simulink model "Simulation_v2"  (R2020a)
settings: Solver=VariableStepAuto  StartTime=0.0  StopTime=tmax  RelTol=1e-3
values from neighbouring files (symbols this model uses):
  BPden = [1 alpha]    [RunSimulation.m]    (also in RunTest.m)
  BPnum = [0.3 alpha]    [RunSimulation.m]    (also in RunTest.m)
  c = 250    [RunSimulation.m]    (also in RunTest.m)
  fc = 0.45    [RunTest.m]
  Ft = 360000    [RunTest.m]
  l = 18    [RunSimulation.m]    (also in RunTest.m)
  num_wagons = 10    [RunTest.m]
  p0 = 0    [RunSimulation.m]    (also in RunTest.m)
  pool = readmatrix('pool.csv')    [RunTest.m]
  Pres = 0/1000*[5.7/771 0 1.6]    [RunSimulation.m]    (also in RunTest.m)
  RBD = 5    [RunSimulation.m]    (also in RunTest.m)
  tl = .1    (= 0.1)    [RunSimulation.m]    (also in RunTest.m)
  trackgradient = 0    [RunTest.m]
  v0 = 100/3.6    (= 27.7777777778)    [RunSimulation.m]
  VBD = 3.5    [RunSimulation.m]    (also in RunTest.m)
libraries: simulink x43, commrandsrc3 x40
(part 2 of 4)

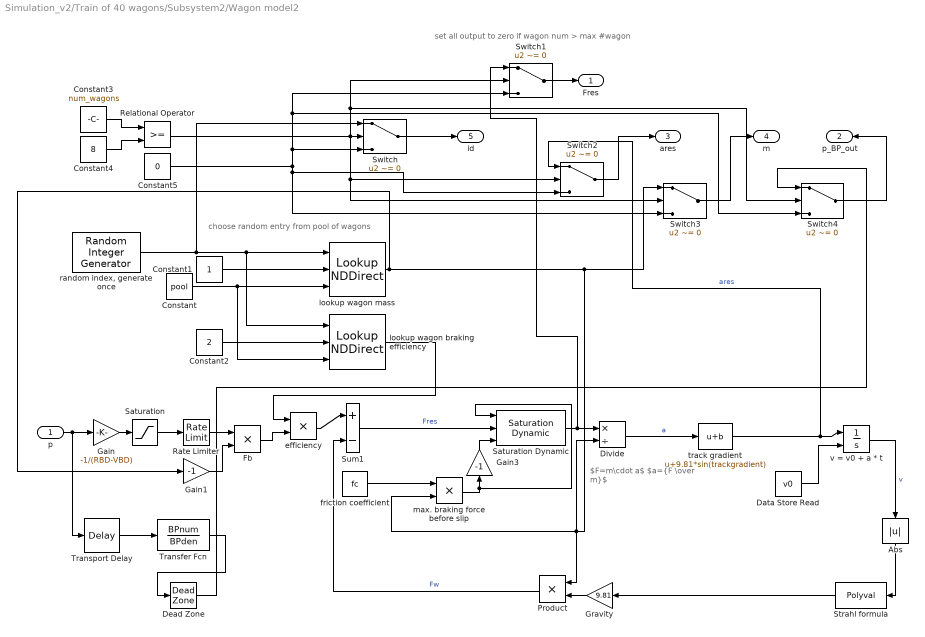
== system Simulation_v2/Train of 40 wagons/Subsystem2/Wagon model2 ==
  note: set all output to zero if wagon num > max #wagon
  note: choose random entry from pool of wagons
  note: $F=m\cdot a$ $a={F \over m}$
  p : Inport
  Abs : Abs
  Constant : Constant  Value=pool
  Constant1 : Constant
  Constant2 : Constant  Value=2
  Constant3 : Constant  Value=num_wagons
  Constant4 : Constant  Value=8
  Constant5 : Constant  Value=0  OutDataTypeStr=uint32
  Data Store Read : DataStoreRead  DataStoreName=v0
  Dead Zone : DeadZone  LowerValue=-0.005  UpperValue=0.005  SaturateOnIntegerOverflow=on
  Divide : Product  Inputs=*/
  Fb : Product  Inputs=**
  Gain : Gain  Gain=-1/(RBD-VBD)
  Gain1 : Gain  Gain=-1
  Gain3 : Gain  Gain=-1
  Gravity : Gain  Gain=9.81
  Product : Product
  Rate Limiter : RateLimiter  RisingSlewLimit=1/tf  FallingSlewLimit=-1/tl  SampleTimeMode=inherited
  Relational Operator : RelationalOperator  OutDataTypeStr=boolean  RndMeth=Simplest
  Saturation : Saturate  UpperLimit=1  LowerLimit=0
  Saturation Dynamic : simulink/Discontinuities/Saturation Dynamic  OutMin=[]  OutMax=[]  OutDataTypeStr=Inherit: Same as second input  OutDataType=fixdt(1, 16)  OutScaling=2^-10  DoSatur=off
  Strahl formula : Polyval  Coefs=Pres
  Sum1 : Sum  Inputs=|+-
  Switch{,1..4} (5 alike) : Switch  Criteria=u2 ~= 0
  Transfer Fcn : TransferFcn  Numerator=BPnum  Denominator=BPden
  Transport Delay : TransportDelay  DelayTime=l/c  InitialOutput=p0
  efficiency : Product  Inputs=**
  friction coefficient : Constant  Value=fc
  lookup wagon braking efficiency : LookupNDDirect  TableIsInput=on
  lookup wagon mass : LookupNDDirect  TableIsInput=on
  max. braking force before slip : Product  Inputs=**
  "random index, generate once " : commrandsrc3/Random Integer Generator  SetSize=500  SeedSource=Auto  Seed=0  SampleTime=999999  SamplesPerFrame=1  OutputDataType=uint32  SimulateUsing=Interpreted execution
  track gradient : Bias  Bias=9.81*sin(trackgradient)
  v = v0 + a * t : Integrator  InitialConditionSource=external  InitialCondition=v0
  Fres : Outport  VectorParamsAs1DForOutWhenUnconnected=off
  p_BP_out : Outport  Port=2  VectorParamsAs1DForOutWhenUnconnected=off
  ares : Outport  Port=3
  m : Outport  Port=4
  "id " : Outport  Port=5
  wires:
  Strahl formula/1 -> Gravity/1
  Abs/1 -> Strahl formula/1
  Gravity/1 -> Product/2
  Product/1 -> Sum1/2  "Fw"
  v = v0 + a * t/1 -> Abs/1  "v"
  lookup wagon mass/1 -> Gain1/1, Switch3/1, max. braking force before slip/2, Divide/2, Product/1
  Divide/1 -> track gradient/1  "a"
  Gain/1 -> Saturation/1
  Fb/1 -> efficiency/2
  Saturation/1 -> Rate Limiter/1
  Rate Limiter/1 -> Fb/1
  Transfer Fcn/1 -> Dead Zone/1
  Transport Delay/1 -> Transfer Fcn/1
  efficiency/1 -> Sum1/1
  track gradient/1 -> Switch2/1, v = v0 + a * t/1  "ares"
  p/1 -> Gain/1, Transport Delay/1
  friction coefficient/1 -> max. braking force before slip/1
  Sum1/1 -> Saturation Dynamic/2  "Fres"
  Saturation Dynamic/1 -> Switch1/1, Divide/1
  max. braking force before slip/1 -> Saturation Dynamic/1, Gain3/1
  Gain3/1 -> Saturation Dynamic/3
  Data Store Read/1 -> v = v0 + a * t/2
  Dead Zone/1 -> Switch4/1
  Constant/1 -> lookup wagon braking efficiency/3, lookup wagon mass/3
  "random index, generate once "/1 -> Switch/1, lookup wagon mass/1, lookup wagon braking efficiency/1
  Constant1/1 -> lookup wagon mass/2
  Constant2/1 -> lookup wagon braking efficiency/2
  lookup wagon braking efficiency/1 -> efficiency/1
  Gain1/1 -> Fb/2
  Constant3/1 -> Relational Operator/1
  Constant4/1 -> Relational Operator/2
  Relational Operator/1 -> Switch1/2, Switch4/2, Switch2/2, Switch3/2, Switch/2
  Switch/1 -> "id "/1
  Constant5/1 -> Switch4/3, Switch1/3, Switch/3, Switch2/3, Switch3/3
  Switch1/1 -> Fres/1
  Switch2/1 -> ares/1
  Switch3/1 -> m/1
  Switch4/1 -> p_BP_out/1

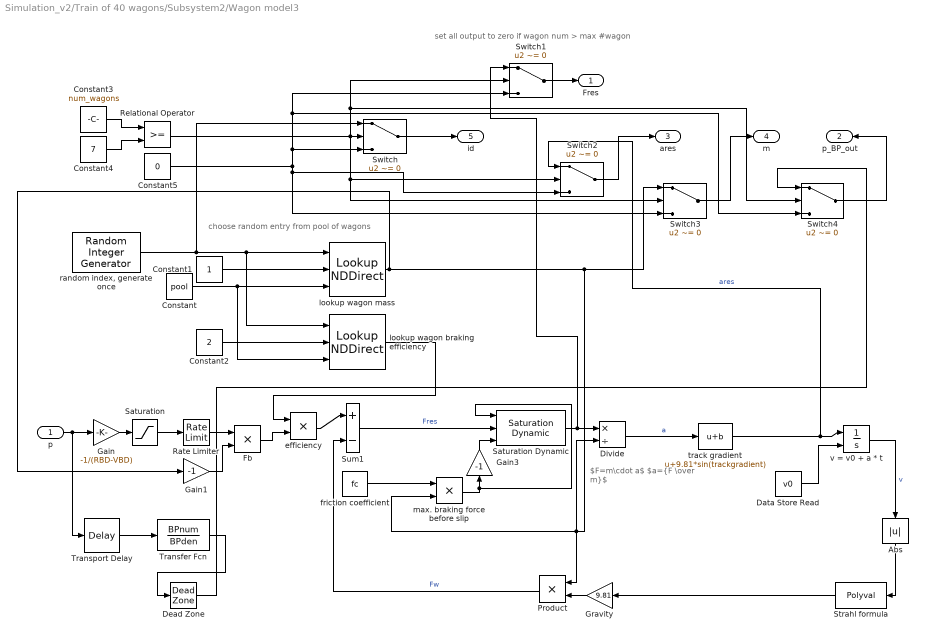
== system Simulation_v2/Train of 40 wagons/Subsystem2/Wagon model3 ==
  note: set all output to zero if wagon num > max #wagon
  note: choose random entry from pool of wagons
  note: $F=m\cdot a$ $a={F \over m}$
  p : Inport
  Abs : Abs
  Constant : Constant  Value=pool
  Constant1 : Constant
  Constant2 : Constant  Value=2
  Constant3 : Constant  Value=num_wagons
  Constant4 : Constant  Value=7
  Constant5 : Constant  Value=0  OutDataTypeStr=uint32
  Data Store Read : DataStoreRead  DataStoreName=v0
  Dead Zone : DeadZone  LowerValue=-0.005  UpperValue=0.005  SaturateOnIntegerOverflow=on
  Divide : Product  Inputs=*/
  Fb : Product  Inputs=**
  Gain : Gain  Gain=-1/(RBD-VBD)
  Gain1 : Gain  Gain=-1
  Gain3 : Gain  Gain=-1
  Gravity : Gain  Gain=9.81
  Product : Product
  Rate Limiter : RateLimiter  RisingSlewLimit=1/tf  FallingSlewLimit=-1/tl  SampleTimeMode=inherited
  Relational Operator : RelationalOperator  OutDataTypeStr=boolean  RndMeth=Simplest
  Saturation : Saturate  UpperLimit=1  LowerLimit=0
  Saturation Dynamic : simulink/Discontinuities/Saturation Dynamic  OutMin=[]  OutMax=[]  OutDataTypeStr=Inherit: Same as second input  OutDataType=fixdt(1, 16)  OutScaling=2^-10  DoSatur=off
  Strahl formula : Polyval  Coefs=Pres
  Sum1 : Sum  Inputs=|+-
  Switch{,1..4} (5 alike) : Switch  Criteria=u2 ~= 0
  Transfer Fcn : TransferFcn  Numerator=BPnum  Denominator=BPden
  Transport Delay : TransportDelay  DelayTime=l/c  InitialOutput=p0
  efficiency : Product  Inputs=**
  friction coefficient : Constant  Value=fc
  lookup wagon braking efficiency : LookupNDDirect  TableIsInput=on
  lookup wagon mass : LookupNDDirect  TableIsInput=on
  max. braking force before slip : Product  Inputs=**
  "random index, generate once " : commrandsrc3/Random Integer Generator  SetSize=500  SeedSource=Auto  Seed=0  SampleTime=999999  SamplesPerFrame=1  OutputDataType=uint32  SimulateUsing=Interpreted execution
  track gradient : Bias  Bias=9.81*sin(trackgradient)
  v = v0 + a * t : Integrator  InitialConditionSource=external  InitialCondition=v0
  Fres : Outport  VectorParamsAs1DForOutWhenUnconnected=off
  p_BP_out : Outport  Port=2  VectorParamsAs1DForOutWhenUnconnected=off
  ares : Outport  Port=3
  m : Outport  Port=4
  "id " : Outport  Port=5
  wires:
  Strahl formula/1 -> Gravity/1
  Abs/1 -> Strahl formula/1
  Gravity/1 -> Product/2
  Product/1 -> Sum1/2  "Fw"
  v = v0 + a * t/1 -> Abs/1  "v"
  lookup wagon mass/1 -> Gain1/1, Switch3/1, max. braking force before slip/2, Divide/2, Product/1
  Divide/1 -> track gradient/1  "a"
  Gain/1 -> Saturation/1
  Fb/1 -> efficiency/2
  Saturation/1 -> Rate Limiter/1
  Rate Limiter/1 -> Fb/1
  Transfer Fcn/1 -> Dead Zone/1
  Transport Delay/1 -> Transfer Fcn/1
  efficiency/1 -> Sum1/1
  track gradient/1 -> Switch2/1, v = v0 + a * t/1  "ares"
  p/1 -> Gain/1, Transport Delay/1
  friction coefficient/1 -> max. braking force before slip/1
  Sum1/1 -> Saturation Dynamic/2  "Fres"
  Saturation Dynamic/1 -> Switch1/1, Divide/1
  max. braking force before slip/1 -> Saturation Dynamic/1, Gain3/1
  Gain3/1 -> Saturation Dynamic/3
  Data Store Read/1 -> v = v0 + a * t/2
  Dead Zone/1 -> Switch4/1
  Constant/1 -> lookup wagon braking efficiency/3, lookup wagon mass/3
  "random index, generate once "/1 -> Switch/1, lookup wagon mass/1, lookup wagon braking efficiency/1
  Constant1/1 -> lookup wagon mass/2
  Constant2/1 -> lookup wagon braking efficiency/2
  lookup wagon braking efficiency/1 -> efficiency/1
  Gain1/1 -> Fb/2
  Constant3/1 -> Relational Operator/1
  Constant4/1 -> Relational Operator/2
  Relational Operator/1 -> Switch1/2, Switch4/2, Switch2/2, Switch3/2, Switch/2
  Switch/1 -> "id "/1
  Constant5/1 -> Switch4/3, Switch1/3, Switch/3, Switch2/3, Switch3/3
  Switch1/1 -> Fres/1
  Switch2/1 -> ares/1
  Switch3/1 -> m/1
  Switch4/1 -> p_BP_out/1

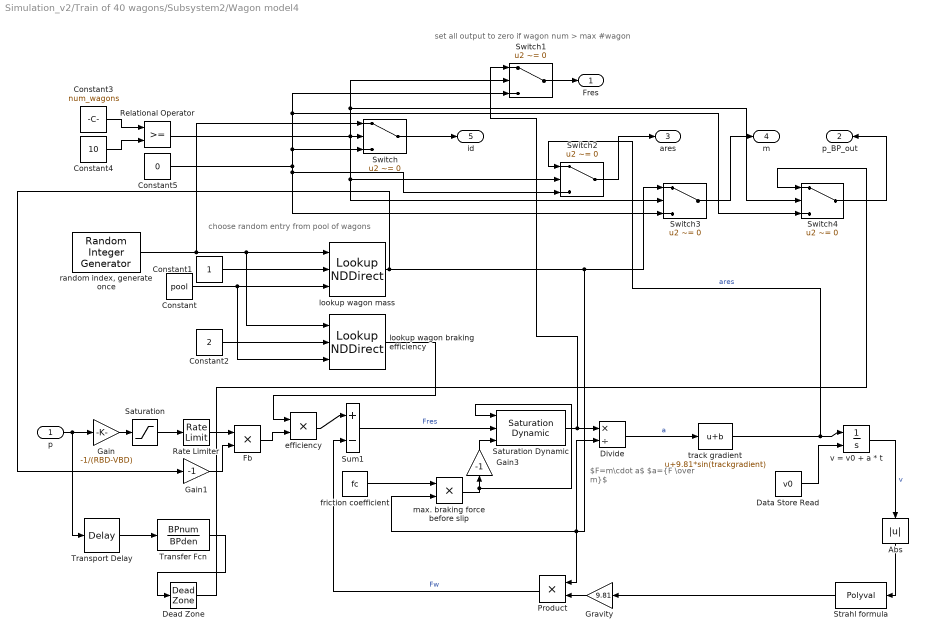
== system Simulation_v2/Train of 40 wagons/Subsystem2/Wagon model4 ==
  note: set all output to zero if wagon num > max #wagon
  note: choose random entry from pool of wagons
  note: $F=m\cdot a$ $a={F \over m}$
  p : Inport
  Abs : Abs
  Constant : Constant  Value=pool
  Constant1 : Constant
  Constant2 : Constant  Value=2
  Constant3 : Constant  Value=num_wagons
  Constant4 : Constant  Value=10
  Constant5 : Constant  Value=0  OutDataTypeStr=uint32
  Data Store Read : DataStoreRead  DataStoreName=v0
  Dead Zone : DeadZone  LowerValue=-0.005  UpperValue=0.005  SaturateOnIntegerOverflow=on
  Divide : Product  Inputs=*/
  Fb : Product  Inputs=**
  Gain : Gain  Gain=-1/(RBD-VBD)
  Gain1 : Gain  Gain=-1
  Gain3 : Gain  Gain=-1
  Gravity : Gain  Gain=9.81
  Product : Product
  Rate Limiter : RateLimiter  RisingSlewLimit=1/tf  FallingSlewLimit=-1/tl  SampleTimeMode=inherited
  Relational Operator : RelationalOperator  OutDataTypeStr=boolean  RndMeth=Simplest
  Saturation : Saturate  UpperLimit=1  LowerLimit=0
  Saturation Dynamic : simulink/Discontinuities/Saturation Dynamic  OutMin=[]  OutMax=[]  OutDataTypeStr=Inherit: Same as second input  OutDataType=fixdt(1, 16)  OutScaling=2^-10  DoSatur=off
  Strahl formula : Polyval  Coefs=Pres
  Sum1 : Sum  Inputs=|+-
  Switch{,1..4} (5 alike) : Switch  Criteria=u2 ~= 0
  Transfer Fcn : TransferFcn  Numerator=BPnum  Denominator=BPden
  Transport Delay : TransportDelay  DelayTime=l/c  InitialOutput=p0
  efficiency : Product  Inputs=**
  friction coefficient : Constant  Value=fc
  lookup wagon braking efficiency : LookupNDDirect  TableIsInput=on
  lookup wagon mass : LookupNDDirect  TableIsInput=on
  max. braking force before slip : Product  Inputs=**
  "random index, generate once " : commrandsrc3/Random Integer Generator  SetSize=500  SeedSource=Auto  Seed=0  SampleTime=999999  SamplesPerFrame=1  OutputDataType=uint32  SimulateUsing=Interpreted execution
  track gradient : Bias  Bias=9.81*sin(trackgradient)
  v = v0 + a * t : Integrator  InitialConditionSource=external  InitialCondition=v0
  Fres : Outport  VectorParamsAs1DForOutWhenUnconnected=off
  p_BP_out : Outport  Port=2  VectorParamsAs1DForOutWhenUnconnected=off
  ares : Outport  Port=3
  m : Outport  Port=4
  "id " : Outport  Port=5
  wires:
  Strahl formula/1 -> Gravity/1
  Abs/1 -> Strahl formula/1
  Gravity/1 -> Product/2
  Product/1 -> Sum1/2  "Fw"
  v = v0 + a * t/1 -> Abs/1  "v"
  lookup wagon mass/1 -> Gain1/1, Switch3/1, max. braking force before slip/2, Divide/2, Product/1
  Divide/1 -> track gradient/1  "a"
  Gain/1 -> Saturation/1
  Fb/1 -> efficiency/2
  Saturation/1 -> Rate Limiter/1
  Rate Limiter/1 -> Fb/1
  Transfer Fcn/1 -> Dead Zone/1
  Transport Delay/1 -> Transfer Fcn/1
  efficiency/1 -> Sum1/1
  track gradient/1 -> Switch2/1, v = v0 + a * t/1  "ares"
  p/1 -> Gain/1, Transport Delay/1
  friction coefficient/1 -> max. braking force before slip/1
  Sum1/1 -> Saturation Dynamic/2  "Fres"
  Saturation Dynamic/1 -> Switch1/1, Divide/1
  max. braking force before slip/1 -> Saturation Dynamic/1, Gain3/1
  Gain3/1 -> Saturation Dynamic/3
  Data Store Read/1 -> v = v0 + a * t/2
  Dead Zone/1 -> Switch4/1
  Constant/1 -> lookup wagon braking efficiency/3, lookup wagon mass/3
  "random index, generate once "/1 -> Switch/1, lookup wagon mass/1, lookup wagon braking efficiency/1
  Constant1/1 -> lookup wagon mass/2
  Constant2/1 -> lookup wagon braking efficiency/2
  lookup wagon braking efficiency/1 -> efficiency/1
  Gain1/1 -> Fb/2
  Constant3/1 -> Relational Operator/1
  Constant4/1 -> Relational Operator/2
  Relational Operator/1 -> Switch1/2, Switch4/2, Switch2/2, Switch3/2, Switch/2
  Switch/1 -> "id "/1
  Constant5/1 -> Switch4/3, Switch1/3, Switch/3, Switch2/3, Switch3/3
  Switch1/1 -> Fres/1
  Switch2/1 -> ares/1
  Switch3/1 -> m/1
  Switch4/1 -> p_BP_out/1

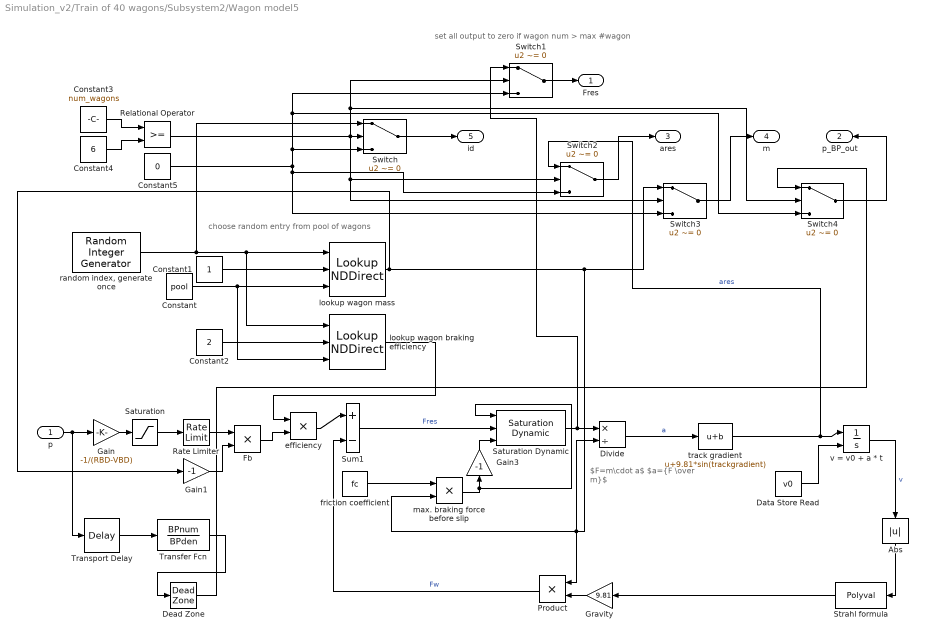
== system Simulation_v2/Train of 40 wagons/Subsystem2/Wagon model5 ==
  note: set all output to zero if wagon num > max #wagon
  note: choose random entry from pool of wagons
  note: $F=m\cdot a$ $a={F \over m}$
  p : Inport
  Abs : Abs
  Constant : Constant  Value=pool
  Constant1 : Constant
  Constant2 : Constant  Value=2
  Constant3 : Constant  Value=num_wagons
  Constant4 : Constant  Value=6
  Constant5 : Constant  Value=0  OutDataTypeStr=uint32
  Data Store Read : DataStoreRead  DataStoreName=v0
  Dead Zone : DeadZone  LowerValue=-0.005  UpperValue=0.005  SaturateOnIntegerOverflow=on
  Divide : Product  Inputs=*/
  Fb : Product  Inputs=**
  Gain : Gain  Gain=-1/(RBD-VBD)
  Gain1 : Gain  Gain=-1
  Gain3 : Gain  Gain=-1
  Gravity : Gain  Gain=9.81
  Product : Product
  Rate Limiter : RateLimiter  RisingSlewLimit=1/tf  FallingSlewLimit=-1/tl  SampleTimeMode=inherited
  Relational Operator : RelationalOperator  OutDataTypeStr=boolean  RndMeth=Simplest
  Saturation : Saturate  UpperLimit=1  LowerLimit=0
  Saturation Dynamic : simulink/Discontinuities/Saturation Dynamic  OutMin=[]  OutMax=[]  OutDataTypeStr=Inherit: Same as second input  OutDataType=fixdt(1, 16)  OutScaling=2^-10  DoSatur=off
  Strahl formula : Polyval  Coefs=Pres
  Sum1 : Sum  Inputs=|+-
  Switch{,1..4} (5 alike) : Switch  Criteria=u2 ~= 0
  Transfer Fcn : TransferFcn  Numerator=BPnum  Denominator=BPden
  Transport Delay : TransportDelay  DelayTime=l/c  InitialOutput=p0
  efficiency : Product  Inputs=**
  friction coefficient : Constant  Value=fc
  lookup wagon braking efficiency : LookupNDDirect  TableIsInput=on
  lookup wagon mass : LookupNDDirect  TableIsInput=on
  max. braking force before slip : Product  Inputs=**
  "random index, generate once " : commrandsrc3/Random Integer Generator  SetSize=500  SeedSource=Auto  Seed=0  SampleTime=999999  SamplesPerFrame=1  OutputDataType=uint32  SimulateUsing=Interpreted execution
  track gradient : Bias  Bias=9.81*sin(trackgradient)
  v = v0 + a * t : Integrator  InitialConditionSource=external  InitialCondition=v0
  Fres : Outport  VectorParamsAs1DForOutWhenUnconnected=off
  p_BP_out : Outport  Port=2  VectorParamsAs1DForOutWhenUnconnected=off
  ares : Outport  Port=3
  m : Outport  Port=4
  "id " : Outport  Port=5
  wires:
  Strahl formula/1 -> Gravity/1
  Abs/1 -> Strahl formula/1
  Gravity/1 -> Product/2
  Product/1 -> Sum1/2  "Fw"
  v = v0 + a * t/1 -> Abs/1  "v"
  lookup wagon mass/1 -> Gain1/1, Switch3/1, max. braking force before slip/2, Divide/2, Product/1
  Divide/1 -> track gradient/1  "a"
  Gain/1 -> Saturation/1
  Fb/1 -> efficiency/2
  Saturation/1 -> Rate Limiter/1
  Rate Limiter/1 -> Fb/1
  Transfer Fcn/1 -> Dead Zone/1
  Transport Delay/1 -> Transfer Fcn/1
  efficiency/1 -> Sum1/1
  track gradient/1 -> Switch2/1, v = v0 + a * t/1  "ares"
  p/1 -> Gain/1, Transport Delay/1
  friction coefficient/1 -> max. braking force before slip/1
  Sum1/1 -> Saturation Dynamic/2  "Fres"
  Saturation Dynamic/1 -> Switch1/1, Divide/1
  max. braking force before slip/1 -> Saturation Dynamic/1, Gain3/1
  Gain3/1 -> Saturation Dynamic/3
  Data Store Read/1 -> v = v0 + a * t/2
  Dead Zone/1 -> Switch4/1
  Constant/1 -> lookup wagon braking efficiency/3, lookup wagon mass/3
  "random index, generate once "/1 -> Switch/1, lookup wagon mass/1, lookup wagon braking efficiency/1
  Constant1/1 -> lookup wagon mass/2
  Constant2/1 -> lookup wagon braking efficiency/2
  lookup wagon braking efficiency/1 -> efficiency/1
  Gain1/1 -> Fb/2
  Constant3/1 -> Relational Operator/1
  Constant4/1 -> Relational Operator/2
  Relational Operator/1 -> Switch1/2, Switch4/2, Switch2/2, Switch3/2, Switch/2
  Switch/1 -> "id "/1
  Constant5/1 -> Switch4/3, Switch1/3, Switch/3, Switch2/3, Switch3/3
  Switch1/1 -> Fres/1
  Switch2/1 -> ares/1
  Switch3/1 -> m/1
  Switch4/1 -> p_BP_out/1

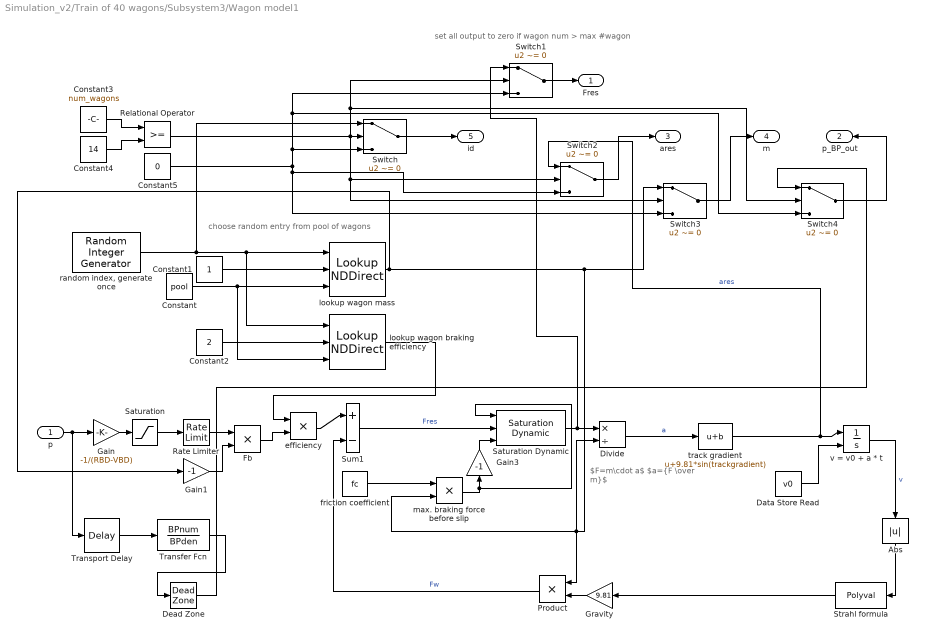
== system Simulation_v2/Train of 40 wagons/Subsystem3/Wagon model1 ==
  note: set all output to zero if wagon num > max #wagon
  note: choose random entry from pool of wagons
  note: $F=m\cdot a$ $a={F \over m}$
  p : Inport
  Abs : Abs
  Constant : Constant  Value=pool
  Constant1 : Constant
  Constant2 : Constant  Value=2
  Constant3 : Constant  Value=num_wagons
  Constant4 : Constant  Value=14
  Constant5 : Constant  Value=0  OutDataTypeStr=uint32
  Data Store Read : DataStoreRead  DataStoreName=v0
  Dead Zone : DeadZone  LowerValue=-0.005  UpperValue=0.005  SaturateOnIntegerOverflow=on
  Divide : Product  Inputs=*/
  Fb : Product  Inputs=**
  Gain : Gain  Gain=-1/(RBD-VBD)
  Gain1 : Gain  Gain=-1
  Gain3 : Gain  Gain=-1
  Gravity : Gain  Gain=9.81
  Product : Product
  Rate Limiter : RateLimiter  RisingSlewLimit=1/tf  FallingSlewLimit=-1/tl  SampleTimeMode=inherited
  Relational Operator : RelationalOperator  OutDataTypeStr=boolean  RndMeth=Simplest
  Saturation : Saturate  UpperLimit=1  LowerLimit=0
  Saturation Dynamic : simulink/Discontinuities/Saturation Dynamic  OutMin=[]  OutMax=[]  OutDataTypeStr=Inherit: Same as second input  OutDataType=fixdt(1, 16)  OutScaling=2^-10  DoSatur=off
  Strahl formula : Polyval  Coefs=Pres
  Sum1 : Sum  Inputs=|+-
  Switch{,1..4} (5 alike) : Switch  Criteria=u2 ~= 0
  Transfer Fcn : TransferFcn  Numerator=BPnum  Denominator=BPden
  Transport Delay : TransportDelay  DelayTime=l/c  InitialOutput=p0
  efficiency : Product  Inputs=**
  friction coefficient : Constant  Value=fc
  lookup wagon braking efficiency : LookupNDDirect  TableIsInput=on
  lookup wagon mass : LookupNDDirect  TableIsInput=on
  max. braking force before slip : Product  Inputs=**
  "random index, generate once " : commrandsrc3/Random Integer Generator  SetSize=500  SeedSource=Auto  Seed=0  SampleTime=999999  SamplesPerFrame=1  OutputDataType=uint32  SimulateUsing=Interpreted execution
  track gradient : Bias  Bias=9.81*sin(trackgradient)
  v = v0 + a * t : Integrator  InitialConditionSource=external  InitialCondition=v0
  Fres : Outport  VectorParamsAs1DForOutWhenUnconnected=off
  p_BP_out : Outport  Port=2  VectorParamsAs1DForOutWhenUnconnected=off
  ares : Outport  Port=3
  m : Outport  Port=4
  "id " : Outport  Port=5
  wires:
  Strahl formula/1 -> Gravity/1
  Abs/1 -> Strahl formula/1
  Gravity/1 -> Product/2
  Product/1 -> Sum1/2  "Fw"
  v = v0 + a * t/1 -> Abs/1  "v"
  lookup wagon mass/1 -> Gain1/1, Switch3/1, max. braking force before slip/2, Divide/2, Product/1
  Divide/1 -> track gradient/1  "a"
  Gain/1 -> Saturation/1
  Fb/1 -> efficiency/2
  Saturation/1 -> Rate Limiter/1
  Rate Limiter/1 -> Fb/1
  Transfer Fcn/1 -> Dead Zone/1
  Transport Delay/1 -> Transfer Fcn/1
  efficiency/1 -> Sum1/1
  track gradient/1 -> Switch2/1, v = v0 + a * t/1  "ares"
  p/1 -> Gain/1, Transport Delay/1
  friction coefficient/1 -> max. braking force before slip/1
  Sum1/1 -> Saturation Dynamic/2  "Fres"
  Saturation Dynamic/1 -> Switch1/1, Divide/1
  max. braking force before slip/1 -> Saturation Dynamic/1, Gain3/1
  Gain3/1 -> Saturation Dynamic/3
  Data Store Read/1 -> v = v0 + a * t/2
  Dead Zone/1 -> Switch4/1
  Constant/1 -> lookup wagon braking efficiency/3, lookup wagon mass/3
  "random index, generate once "/1 -> Switch/1, lookup wagon mass/1, lookup wagon braking efficiency/1
  Constant1/1 -> lookup wagon mass/2
  Constant2/1 -> lookup wagon braking efficiency/2
  lookup wagon braking efficiency/1 -> efficiency/1
  Gain1/1 -> Fb/2
  Constant3/1 -> Relational Operator/1
  Constant4/1 -> Relational Operator/2
  Relational Operator/1 -> Switch1/2, Switch4/2, Switch2/2, Switch3/2, Switch/2
  Switch/1 -> "id "/1
  Constant5/1 -> Switch4/3, Switch1/3, Switch/3, Switch2/3, Switch3/3
  Switch1/1 -> Fres/1
  Switch2/1 -> ares/1
  Switch3/1 -> m/1
  Switch4/1 -> p_BP_out/1

== system Simulation_v2/Train of 40 wagons/Subsystem3/Wagon model2 ==
  note: set all output to zero if wagon num > max #wagon
  note: choose random entry from pool of wagons
  note: $F=m\cdot a$ $a={F \over m}$
  p : Inport
  Abs : Abs
  Constant : Constant  Value=pool
  Constant1 : Constant
  Constant2 : Constant  Value=2
  Constant3 : Constant  Value=num_wagons
  Constant4 : Constant  Value=13
  Constant5 : Constant  Value=0  OutDataTypeStr=uint32
  Data Store Read : DataStoreRead  DataStoreName=v0
  Dead Zone : DeadZone  LowerValue=-0.005  UpperValue=0.005  SaturateOnIntegerOverflow=on
  Divide : Product  Inputs=*/
  Fb : Product  Inputs=**
  Gain : Gain  Gain=-1/(RBD-VBD)
  Gain1 : Gain  Gain=-1
  Gain3 : Gain  Gain=-1
  Gravity : Gain  Gain=9.81
  Product : Product
  Rate Limiter : RateLimiter  RisingSlewLimit=1/tf  FallingSlewLimit=-1/tl  SampleTimeMode=inherited
  Relational Operator : RelationalOperator  OutDataTypeStr=boolean  RndMeth=Simplest
  Saturation : Saturate  UpperLimit=1  LowerLimit=0
  Saturation Dynamic : simulink/Discontinuities/Saturation Dynamic  OutMin=[]  OutMax=[]  OutDataTypeStr=Inherit: Same as second input  OutDataType=fixdt(1, 16)  OutScaling=2^-10  DoSatur=off
  Strahl formula : Polyval  Coefs=Pres
  Sum1 : Sum  Inputs=|+-
  Switch{,1..4} (5 alike) : Switch  Criteria=u2 ~= 0
  Transfer Fcn : TransferFcn  Numerator=BPnum  Denominator=BPden
  Transport Delay : TransportDelay  DelayTime=l/c  InitialOutput=p0
  efficiency : Product  Inputs=**
  friction coefficient : Constant  Value=fc
  lookup wagon braking efficiency : LookupNDDirect  TableIsInput=on
  lookup wagon mass : LookupNDDirect  TableIsInput=on
  max. braking force before slip : Product  Inputs=**
  "random index, generate once " : commrandsrc3/Random Integer Generator  SetSize=500  SeedSource=Auto  Seed=0  SampleTime=999999  SamplesPerFrame=1  OutputDataType=uint32  SimulateUsing=Interpreted execution
  track gradient : Bias  Bias=9.81*sin(trackgradient)
  v = v0 + a * t : Integrator  InitialConditionSource=external  InitialCondition=v0
  Fres : Outport  VectorParamsAs1DForOutWhenUnconnected=off
  p_BP_out : Outport  Port=2  VectorParamsAs1DForOutWhenUnconnected=off
  ares : Outport  Port=3
  m : Outport  Port=4
  "id " : Outport  Port=5
  wires:
  Strahl formula/1 -> Gravity/1
  Abs/1 -> Strahl formula/1
  Gravity/1 -> Product/2
  Product/1 -> Sum1/2  "Fw"
  v = v0 + a * t/1 -> Abs/1  "v"
  lookup wagon mass/1 -> Gain1/1, Switch3/1, max. braking force before slip/2, Divide/2, Product/1
  Divide/1 -> track gradient/1  "a"
  Gain/1 -> Saturation/1
  Fb/1 -> efficiency/2
  Saturation/1 -> Rate Limiter/1
  Rate Limiter/1 -> Fb/1
  Transfer Fcn/1 -> Dead Zone/1
  Transport Delay/1 -> Transfer Fcn/1
  efficiency/1 -> Sum1/1
  track gradient/1 -> Switch2/1, v = v0 + a * t/1  "ares"
  p/1 -> Gain/1, Transport Delay/1
  friction coefficient/1 -> max. braking force before slip/1
  Sum1/1 -> Saturation Dynamic/2  "Fres"
  Saturation Dynamic/1 -> Switch1/1, Divide/1
  max. braking force before slip/1 -> Saturation Dynamic/1, Gain3/1
  Gain3/1 -> Saturation Dynamic/3
  Data Store Read/1 -> v = v0 + a * t/2
  Dead Zone/1 -> Switch4/1
  Constant/1 -> lookup wagon braking efficiency/3, lookup wagon mass/3
  "random index, generate once "/1 -> Switch/1, lookup wagon mass/1, lookup wagon braking efficiency/1
  Constant1/1 -> lookup wagon mass/2
  Constant2/1 -> lookup wagon braking efficiency/2
  lookup wagon braking efficiency/1 -> efficiency/1
  Gain1/1 -> Fb/2
  Constant3/1 -> Relational Operator/1
  Constant4/1 -> Relational Operator/2
  Relational Operator/1 -> Switch1/2, Switch4/2, Switch2/2, Switch3/2, Switch/2
  Switch/1 -> "id "/1
  Constant5/1 -> Switch4/3, Switch1/3, Switch/3, Switch2/3, Switch3/3
  Switch1/1 -> Fres/1
  Switch2/1 -> ares/1
  Switch3/1 -> m/1
  Switch4/1 -> p_BP_out/1

== system Simulation_v2/Train of 40 wagons/Subsystem3/Wagon model3 ==
  note: set all output to zero if wagon num > max #wagon
  note: choose random entry from pool of wagons
  note: $F=m\cdot a$ $a={F \over m}$
  p : Inport
  Abs : Abs
  Constant : Constant  Value=pool
  Constant1 : Constant
  Constant2 : Constant  Value=2
  Constant3 : Constant  Value=num_wagons
  Constant4 : Constant  Value=12
  Constant5 : Constant  Value=0  OutDataTypeStr=uint32
  Data Store Read : DataStoreRead  DataStoreName=v0
  Dead Zone : DeadZone  LowerValue=-0.005  UpperValue=0.005  SaturateOnIntegerOverflow=on
  Divide : Product  Inputs=*/
  Fb : Product  Inputs=**
  Gain : Gain  Gain=-1/(RBD-VBD)
  Gain1 : Gain  Gain=-1
  Gain3 : Gain  Gain=-1
  Gravity : Gain  Gain=9.81
  Product : Product
  Rate Limiter : RateLimiter  RisingSlewLimit=1/tf  FallingSlewLimit=-1/tl  SampleTimeMode=inherited
  Relational Operator : RelationalOperator  OutDataTypeStr=boolean  RndMeth=Simplest
  Saturation : Saturate  UpperLimit=1  LowerLimit=0
  Saturation Dynamic : simulink/Discontinuities/Saturation Dynamic  OutMin=[]  OutMax=[]  OutDataTypeStr=Inherit: Same as second input  OutDataType=fixdt(1, 16)  OutScaling=2^-10  DoSatur=off
  Strahl formula : Polyval  Coefs=Pres
  Sum1 : Sum  Inputs=|+-
  Switch{,1..4} (5 alike) : Switch  Criteria=u2 ~= 0
  Transfer Fcn : TransferFcn  Numerator=BPnum  Denominator=BPden
  Transport Delay : TransportDelay  DelayTime=l/c  InitialOutput=p0
  efficiency : Product  Inputs=**
  friction coefficient : Constant  Value=fc
  lookup wagon braking efficiency : LookupNDDirect  TableIsInput=on
  lookup wagon mass : LookupNDDirect  TableIsInput=on
  max. braking force before slip : Product  Inputs=**
  "random index, generate once " : commrandsrc3/Random Integer Generator  SetSize=500  SeedSource=Auto  Seed=0  SampleTime=999999  SamplesPerFrame=1  OutputDataType=uint32  SimulateUsing=Interpreted execution
  track gradient : Bias  Bias=9.81*sin(trackgradient)
  v = v0 + a * t : Integrator  InitialConditionSource=external  InitialCondition=v0
  Fres : Outport  VectorParamsAs1DForOutWhenUnconnected=off
  p_BP_out : Outport  Port=2  VectorParamsAs1DForOutWhenUnconnected=off
  ares : Outport  Port=3
  m : Outport  Port=4
  "id " : Outport  Port=5
  wires:
  Strahl formula/1 -> Gravity/1
  Abs/1 -> Strahl formula/1
  Gravity/1 -> Product/2
  Product/1 -> Sum1/2  "Fw"
  v = v0 + a * t/1 -> Abs/1  "v"
  lookup wagon mass/1 -> Gain1/1, Switch3/1, max. braking force before slip/2, Divide/2, Product/1
  Divide/1 -> track gradient/1  "a"
  Gain/1 -> Saturation/1
  Fb/1 -> efficiency/2
  Saturation/1 -> Rate Limiter/1
  Rate Limiter/1 -> Fb/1
  Transfer Fcn/1 -> Dead Zone/1
  Transport Delay/1 -> Transfer Fcn/1
  efficiency/1 -> Sum1/1
  track gradient/1 -> Switch2/1, v = v0 + a * t/1  "ares"
  p/1 -> Gain/1, Transport Delay/1
  friction coefficient/1 -> max. braking force before slip/1
  Sum1/1 -> Saturation Dynamic/2  "Fres"
  Saturation Dynamic/1 -> Switch1/1, Divide/1
  max. braking force before slip/1 -> Saturation Dynamic/1, Gain3/1
  Gain3/1 -> Saturation Dynamic/3
  Data Store Read/1 -> v = v0 + a * t/2
  Dead Zone/1 -> Switch4/1
  Constant/1 -> lookup wagon braking efficiency/3, lookup wagon mass/3
  "random index, generate once "/1 -> Switch/1, lookup wagon mass/1, lookup wagon braking efficiency/1
  Constant1/1 -> lookup wagon mass/2
  Constant2/1 -> lookup wagon braking efficiency/2
  lookup wagon braking efficiency/1 -> efficiency/1
  Gain1/1 -> Fb/2
  Constant3/1 -> Relational Operator/1
  Constant4/1 -> Relational Operator/2
  Relational Operator/1 -> Switch1/2, Switch4/2, Switch2/2, Switch3/2, Switch/2
  Switch/1 -> "id "/1
  Constant5/1 -> Switch4/3, Switch1/3, Switch/3, Switch2/3, Switch3/3
  Switch1/1 -> Fres/1
  Switch2/1 -> ares/1
  Switch3/1 -> m/1
  Switch4/1 -> p_BP_out/1

== system Simulation_v2/Train of 40 wagons/Subsystem3/Wagon model4 ==
  note: set all output to zero if wagon num > max #wagon
  note: choose random entry from pool of wagons
  note: $F=m\cdot a$ $a={F \over m}$
  p : Inport
  Abs : Abs
  Constant : Constant  Value=pool
  Constant1 : Constant
  Constant2 : Constant  Value=2
  Constant3 : Constant  Value=num_wagons
  Constant4 : Constant  Value=15
  Constant5 : Constant  Value=0  OutDataTypeStr=uint32
  Data Store Read : DataStoreRead  DataStoreName=v0
  Dead Zone : DeadZone  LowerValue=-0.005  UpperValue=0.005  SaturateOnIntegerOverflow=on
  Divide : Product  Inputs=*/
  Fb : Product  Inputs=**
  Gain : Gain  Gain=-1/(RBD-VBD)
  Gain1 : Gain  Gain=-1
  Gain3 : Gain  Gain=-1
  Gravity : Gain  Gain=9.81
  Product : Product
  Rate Limiter : RateLimiter  RisingSlewLimit=1/tf  FallingSlewLimit=-1/tl  SampleTimeMode=inherited
  Relational Operator : RelationalOperator  OutDataTypeStr=boolean  RndMeth=Simplest
  Saturation : Saturate  UpperLimit=1  LowerLimit=0
  Saturation Dynamic : simulink/Discontinuities/Saturation Dynamic  OutMin=[]  OutMax=[]  OutDataTypeStr=Inherit: Same as second input  OutDataType=fixdt(1, 16)  OutScaling=2^-10  DoSatur=off
  Strahl formula : Polyval  Coefs=Pres
  Sum1 : Sum  Inputs=|+-
  Switch{,1..4} (5 alike) : Switch  Criteria=u2 ~= 0
  Transfer Fcn : TransferFcn  Numerator=BPnum  Denominator=BPden
  Transport Delay : TransportDelay  DelayTime=l/c  InitialOutput=p0
  efficiency : Product  Inputs=**
  friction coefficient : Constant  Value=fc
  lookup wagon braking efficiency : LookupNDDirect  TableIsInput=on
  lookup wagon mass : LookupNDDirect  TableIsInput=on
  max. braking force before slip : Product  Inputs=**
  "random index, generate once " : commrandsrc3/Random Integer Generator  SetSize=500  SeedSource=Auto  Seed=0  SampleTime=999999  SamplesPerFrame=1  OutputDataType=uint32  SimulateUsing=Interpreted execution
  track gradient : Bias  Bias=9.81*sin(trackgradient)
  v = v0 + a * t : Integrator  InitialConditionSource=external  InitialCondition=v0
  Fres : Outport  VectorParamsAs1DForOutWhenUnconnected=off
  p_BP_out : Outport  Port=2  VectorParamsAs1DForOutWhenUnconnected=off
  ares : Outport  Port=3
  m : Outport  Port=4
  "id " : Outport  Port=5
  wires:
  Strahl formula/1 -> Gravity/1
  Abs/1 -> Strahl formula/1
  Gravity/1 -> Product/2
  Product/1 -> Sum1/2  "Fw"
  v = v0 + a * t/1 -> Abs/1  "v"
  lookup wagon mass/1 -> Gain1/1, Switch3/1, max. braking force before slip/2, Divide/2, Product/1
  Divide/1 -> track gradient/1  "a"
  Gain/1 -> Saturation/1
  Fb/1 -> efficiency/2
  Saturation/1 -> Rate Limiter/1
  Rate Limiter/1 -> Fb/1
  Transfer Fcn/1 -> Dead Zone/1
  Transport Delay/1 -> Transfer Fcn/1
  efficiency/1 -> Sum1/1
  track gradient/1 -> Switch2/1, v = v0 + a * t/1  "ares"
  p/1 -> Gain/1, Transport Delay/1
  friction coefficient/1 -> max. braking force before slip/1
  Sum1/1 -> Saturation Dynamic/2  "Fres"
  Saturation Dynamic/1 -> Switch1/1, Divide/1
  max. braking force before slip/1 -> Saturation Dynamic/1, Gain3/1
  Gain3/1 -> Saturation Dynamic/3
  Data Store Read/1 -> v = v0 + a * t/2
  Dead Zone/1 -> Switch4/1
  Constant/1 -> lookup wagon braking efficiency/3, lookup wagon mass/3
  "random index, generate once "/1 -> Switch/1, lookup wagon mass/1, lookup wagon braking efficiency/1
  Constant1/1 -> lookup wagon mass/2
  Constant2/1 -> lookup wagon braking efficiency/2
  lookup wagon braking efficiency/1 -> efficiency/1
  Gain1/1 -> Fb/2
  Constant3/1 -> Relational Operator/1
  Constant4/1 -> Relational Operator/2
  Relational Operator/1 -> Switch1/2, Switch4/2, Switch2/2, Switch3/2, Switch/2
  Switch/1 -> "id "/1
  Constant5/1 -> Switch4/3, Switch1/3, Switch/3, Switch2/3, Switch3/3
  Switch1/1 -> Fres/1
  Switch2/1 -> ares/1
  Switch3/1 -> m/1
  Switch4/1 -> p_BP_out/1

== system Simulation_v2/Train of 40 wagons/Subsystem3/Wagon model5 ==
  note: set all output to zero if wagon num > max #wagon
  note: choose random entry from pool of wagons
  note: $F=m\cdot a$ $a={F \over m}$
  p : Inport
  Abs : Abs
  Constant : Constant  Value=pool
  Constant1 : Constant
  Constant2 : Constant  Value=2
  Constant3 : Constant  Value=num_wagons
  Constant4 : Constant  Value=11
  Constant5 : Constant  Value=0  OutDataTypeStr=uint32
  Data Store Read : DataStoreRead  DataStoreName=v0
  Dead Zone : DeadZone  LowerValue=-0.005  UpperValue=0.005  SaturateOnIntegerOverflow=on
  Divide : Product  Inputs=*/
  Fb : Product  Inputs=**
  Gain : Gain  Gain=-1/(RBD-VBD)
  Gain1 : Gain  Gain=-1
  Gain3 : Gain  Gain=-1
  Gravity : Gain  Gain=9.81
  Product : Product
  Rate Limiter : RateLimiter  RisingSlewLimit=1/tf  FallingSlewLimit=-1/tl  SampleTimeMode=inherited
  Relational Operator : RelationalOperator  OutDataTypeStr=boolean  RndMeth=Simplest
  Saturation : Saturate  UpperLimit=1  LowerLimit=0
  Saturation Dynamic : simulink/Discontinuities/Saturation Dynamic  OutMin=[]  OutMax=[]  OutDataTypeStr=Inherit: Same as second input  OutDataType=fixdt(1, 16)  OutScaling=2^-10  DoSatur=off
  Strahl formula : Polyval  Coefs=Pres
  Sum1 : Sum  Inputs=|+-
  Switch{,1..4} (5 alike) : Switch  Criteria=u2 ~= 0
  Transfer Fcn : TransferFcn  Numerator=BPnum  Denominator=BPden
  Transport Delay : TransportDelay  DelayTime=l/c  InitialOutput=p0
  efficiency : Product  Inputs=**
  friction coefficient : Constant  Value=fc
  lookup wagon braking efficiency : LookupNDDirect  TableIsInput=on
  lookup wagon mass : LookupNDDirect  TableIsInput=on
  max. braking force before slip : Product  Inputs=**
  "random index, generate once " : commrandsrc3/Random Integer Generator  SetSize=500  SeedSource=Auto  Seed=0  SampleTime=999999  SamplesPerFrame=1  OutputDataType=uint32  SimulateUsing=Interpreted execution
  track gradient : Bias  Bias=9.81*sin(trackgradient)
  v = v0 + a * t : Integrator  InitialConditionSource=external  InitialCondition=v0
  Fres : Outport  VectorParamsAs1DForOutWhenUnconnected=off
  p_BP_out : Outport  Port=2  VectorParamsAs1DForOutWhenUnconnected=off
  ares : Outport  Port=3
  m : Outport  Port=4
  "id " : Outport  Port=5
  wires:
  Strahl formula/1 -> Gravity/1
  Abs/1 -> Strahl formula/1
  Gravity/1 -> Product/2
  Product/1 -> Sum1/2  "Fw"
  v = v0 + a * t/1 -> Abs/1  "v"
  lookup wagon mass/1 -> Gain1/1, Switch3/1, max. braking force before slip/2, Divide/2, Product/1
  Divide/1 -> track gradient/1  "a"
  Gain/1 -> Saturation/1
  Fb/1 -> efficiency/2
  Saturation/1 -> Rate Limiter/1
  Rate Limiter/1 -> Fb/1
  Transfer Fcn/1 -> Dead Zone/1
  Transport Delay/1 -> Transfer Fcn/1
  efficiency/1 -> Sum1/1
  track gradient/1 -> Switch2/1, v = v0 + a * t/1  "ares"
  p/1 -> Gain/1, Transport Delay/1
  friction coefficient/1 -> max. braking force before slip/1
  Sum1/1 -> Saturation Dynamic/2  "Fres"
  Saturation Dynamic/1 -> Switch1/1, Divide/1
  max. braking force before slip/1 -> Saturation Dynamic/1, Gain3/1
  Gain3/1 -> Saturation Dynamic/3
  Data Store Read/1 -> v = v0 + a * t/2
  Dead Zone/1 -> Switch4/1
  Constant/1 -> lookup wagon braking efficiency/3, lookup wagon mass/3
  "random index, generate once "/1 -> Switch/1, lookup wagon mass/1, lookup wagon braking efficiency/1
  Constant1/1 -> lookup wagon mass/2
  Constant2/1 -> lookup wagon braking efficiency/2
  lookup wagon braking efficiency/1 -> efficiency/1
  Gain1/1 -> Fb/2
  Constant3/1 -> Relational Operator/1
  Constant4/1 -> Relational Operator/2
  Relational Operator/1 -> Switch1/2, Switch4/2, Switch2/2, Switch3/2, Switch/2
  Switch/1 -> "id "/1
  Constant5/1 -> Switch4/3, Switch1/3, Switch/3, Switch2/3, Switch3/3
  Switch1/1 -> Fres/1
  Switch2/1 -> ares/1
  Switch3/1 -> m/1
  Switch4/1 -> p_BP_out/1

== system Simulation_v2/Train of 40 wagons/Subsystem4/Wagon model1 ==
  note: set all output to zero if wagon num > max #wagon
  note: choose random entry from pool of wagons
  note: $F=m\cdot a$ $a={F \over m}$
  p : Inport
  Abs : Abs
  Constant : Constant  Value=pool
  Constant1 : Constant
  Constant2 : Constant  Value=2
  Constant3 : Constant  Value=num_wagons
  Constant4 : Constant  Value=19
  Constant5 : Constant  Value=0  OutDataTypeStr=uint32
  Data Store Read : DataStoreRead  DataStoreName=v0
  Dead Zone : DeadZone  LowerValue=-0.005  UpperValue=0.005  SaturateOnIntegerOverflow=on
  Divide : Product  Inputs=*/
  Fb : Product  Inputs=**
  Gain : Gain  Gain=-1/(RBD-VBD)
  Gain1 : Gain  Gain=-1
  Gain3 : Gain  Gain=-1
  Gravity : Gain  Gain=9.81
  Product : Product
  Rate Limiter : RateLimiter  RisingSlewLimit=1/tf  FallingSlewLimit=-1/tl  SampleTimeMode=inherited
  Relational Operator : RelationalOperator  OutDataTypeStr=boolean  RndMeth=Simplest
  Saturation : Saturate  UpperLimit=1  LowerLimit=0
  Saturation Dynamic : simulink/Discontinuities/Saturation Dynamic  OutMin=[]  OutMax=[]  OutDataTypeStr=Inherit: Same as second input  OutDataType=fixdt(1, 16)  OutScaling=2^-10  DoSatur=off
  Strahl formula : Polyval  Coefs=Pres
  Sum1 : Sum  Inputs=|+-
  Switch{,1..4} (5 alike) : Switch  Criteria=u2 ~= 0
  Transfer Fcn : TransferFcn  Numerator=BPnum  Denominator=BPden
  Transport Delay : TransportDelay  DelayTime=l/c  InitialOutput=p0
  efficiency : Product  Inputs=**
  friction coefficient : Constant  Value=fc
  lookup wagon braking efficiency : LookupNDDirect  TableIsInput=on
  lookup wagon mass : LookupNDDirect  TableIsInput=on
  max. braking force before slip : Product  Inputs=**
  "random index, generate once " : commrandsrc3/Random Integer Generator  SetSize=500  SeedSource=Auto  Seed=0  SampleTime=999999  SamplesPerFrame=1  OutputDataType=uint32  SimulateUsing=Interpreted execution
  track gradient : Bias  Bias=9.81*sin(trackgradient)
  v = v0 + a * t : Integrator  InitialConditionSource=external  InitialCondition=v0
  Fres : Outport  VectorParamsAs1DForOutWhenUnconnected=off
  p_BP_out : Outport  Port=2  VectorParamsAs1DForOutWhenUnconnected=off
  ares : Outport  Port=3
  m : Outport  Port=4
  "id " : Outport  Port=5
  wires:
  Strahl formula/1 -> Gravity/1
  Abs/1 -> Strahl formula/1
  Gravity/1 -> Product/2
  Product/1 -> Sum1/2  "Fw"
  v = v0 + a * t/1 -> Abs/1  "v"
  lookup wagon mass/1 -> Gain1/1, Switch3/1, max. braking force before slip/2, Divide/2, Product/1
  Divide/1 -> track gradient/1  "a"
  Gain/1 -> Saturation/1
  Fb/1 -> efficiency/2
  Saturation/1 -> Rate Limiter/1
  Rate Limiter/1 -> Fb/1
  Transfer Fcn/1 -> Dead Zone/1
  Transport Delay/1 -> Transfer Fcn/1
  efficiency/1 -> Sum1/1
  track gradient/1 -> Switch2/1, v = v0 + a * t/1  "ares"
  p/1 -> Gain/1, Transport Delay/1
  friction coefficient/1 -> max. braking force before slip/1
  Sum1/1 -> Saturation Dynamic/2  "Fres"
  Saturation Dynamic/1 -> Switch1/1, Divide/1
  max. braking force before slip/1 -> Saturation Dynamic/1, Gain3/1
  Gain3/1 -> Saturation Dynamic/3
  Data Store Read/1 -> v = v0 + a * t/2
  Dead Zone/1 -> Switch4/1
  Constant/1 -> lookup wagon braking efficiency/3, lookup wagon mass/3
  "random index, generate once "/1 -> Switch/1, lookup wagon mass/1, lookup wagon braking efficiency/1
  Constant1/1 -> lookup wagon mass/2
  Constant2/1 -> lookup wagon braking efficiency/2
  lookup wagon braking efficiency/1 -> efficiency/1
  Gain1/1 -> Fb/2
  Constant3/1 -> Relational Operator/1
  Constant4/1 -> Relational Operator/2
  Relational Operator/1 -> Switch1/2, Switch4/2, Switch2/2, Switch3/2, Switch/2
  Switch/1 -> "id "/1
  Constant5/1 -> Switch4/3, Switch1/3, Switch/3, Switch2/3, Switch3/3
  Switch1/1 -> Fres/1
  Switch2/1 -> ares/1
  Switch3/1 -> m/1
  Switch4/1 -> p_BP_out/1

== system Simulation_v2/Train of 40 wagons/Subsystem4/Wagon model2 ==
  note: set all output to zero if wagon num > max #wagon
  note: choose random entry from pool of wagons
  note: $F=m\cdot a$ $a={F \over m}$
  p : Inport
  Abs : Abs
  Constant : Constant  Value=pool
  Constant1 : Constant
  Constant2 : Constant  Value=2
  Constant3 : Constant  Value=num_wagons
  Constant4 : Constant  Value=18
  Constant5 : Constant  Value=0  OutDataTypeStr=uint32
  Data Store Read : DataStoreRead  DataStoreName=v0
  Dead Zone : DeadZone  LowerValue=-0.005  UpperValue=0.005  SaturateOnIntegerOverflow=on
  Divide : Product  Inputs=*/
  Fb : Product  Inputs=**
  Gain : Gain  Gain=-1/(RBD-VBD)
  Gain1 : Gain  Gain=-1
  Gain3 : Gain  Gain=-1
  Gravity : Gain  Gain=9.81
  Product : Product
  Rate Limiter : RateLimiter  RisingSlewLimit=1/tf  FallingSlewLimit=-1/tl  SampleTimeMode=inherited
  Relational Operator : RelationalOperator  OutDataTypeStr=boolean  RndMeth=Simplest
  Saturation : Saturate  UpperLimit=1  LowerLimit=0
  Saturation Dynamic : simulink/Discontinuities/Saturation Dynamic  OutMin=[]  OutMax=[]  OutDataTypeStr=Inherit: Same as second input  OutDataType=fixdt(1, 16)  OutScaling=2^-10  DoSatur=off
  Strahl formula : Polyval  Coefs=Pres
  Sum1 : Sum  Inputs=|+-
  Switch{,1..4} (5 alike) : Switch  Criteria=u2 ~= 0
  Transfer Fcn : TransferFcn  Numerator=BPnum  Denominator=BPden
  Transport Delay : TransportDelay  DelayTime=l/c  InitialOutput=p0
  efficiency : Product  Inputs=**
  friction coefficient : Constant  Value=fc
  lookup wagon braking efficiency : LookupNDDirect  TableIsInput=on
  lookup wagon mass : LookupNDDirect  TableIsInput=on
  max. braking force before slip : Product  Inputs=**
  "random index, generate once " : commrandsrc3/Random Integer Generator  SetSize=500  SeedSource=Auto  Seed=0  SampleTime=999999  SamplesPerFrame=1  OutputDataType=uint32  SimulateUsing=Interpreted execution
  track gradient : Bias  Bias=9.81*sin(trackgradient)
  v = v0 + a * t : Integrator  InitialConditionSource=external  InitialCondition=v0
  Fres : Outport  VectorParamsAs1DForOutWhenUnconnected=off
  p_BP_out : Outport  Port=2  VectorParamsAs1DForOutWhenUnconnected=off
  ares : Outport  Port=3
  m : Outport  Port=4
  "id " : Outport  Port=5
  wires:
  Strahl formula/1 -> Gravity/1
  Abs/1 -> Strahl formula/1
  Gravity/1 -> Product/2
  Product/1 -> Sum1/2  "Fw"
  v = v0 + a * t/1 -> Abs/1  "v"
  lookup wagon mass/1 -> Gain1/1, Switch3/1, max. braking force before slip/2, Divide/2, Product/1
  Divide/1 -> track gradient/1  "a"
  Gain/1 -> Saturation/1
  Fb/1 -> efficiency/2
  Saturation/1 -> Rate Limiter/1
  Rate Limiter/1 -> Fb/1
  Transfer Fcn/1 -> Dead Zone/1
  Transport Delay/1 -> Transfer Fcn/1
  efficiency/1 -> Sum1/1
  track gradient/1 -> Switch2/1, v = v0 + a * t/1  "ares"
  p/1 -> Gain/1, Transport Delay/1
  friction coefficient/1 -> max. braking force before slip/1
  Sum1/1 -> Saturation Dynamic/2  "Fres"
  Saturation Dynamic/1 -> Switch1/1, Divide/1
  max. braking force before slip/1 -> Saturation Dynamic/1, Gain3/1
  Gain3/1 -> Saturation Dynamic/3
  Data Store Read/1 -> v = v0 + a * t/2
  Dead Zone/1 -> Switch4/1
  Constant/1 -> lookup wagon braking efficiency/3, lookup wagon mass/3
  "random index, generate once "/1 -> Switch/1, lookup wagon mass/1, lookup wagon braking efficiency/1
  Constant1/1 -> lookup wagon mass/2
  Constant2/1 -> lookup wagon braking efficiency/2
  lookup wagon braking efficiency/1 -> efficiency/1
  Gain1/1 -> Fb/2
  Constant3/1 -> Relational Operator/1
  Constant4/1 -> Relational Operator/2
  Relational Operator/1 -> Switch1/2, Switch4/2, Switch2/2, Switch3/2, Switch/2
  Switch/1 -> "id "/1
  Constant5/1 -> Switch4/3, Switch1/3, Switch/3, Switch2/3, Switch3/3
  Switch1/1 -> Fres/1
  Switch2/1 -> ares/1
  Switch3/1 -> m/1
  Switch4/1 -> p_BP_out/1

== system Simulation_v2/Train of 40 wagons/Subsystem4/Wagon model3 ==
  note: set all output to zero if wagon num > max #wagon
  note: choose random entry from pool of wagons
  note: $F=m\cdot a$ $a={F \over m}$
  p : Inport
  Abs : Abs
  Constant : Constant  Value=pool
  Constant1 : Constant
  Constant2 : Constant  Value=2
  Constant3 : Constant  Value=num_wagons
  Constant4 : Constant  Value=17
  Constant5 : Constant  Value=0  OutDataTypeStr=uint32
  Data Store Read : DataStoreRead  DataStoreName=v0
  Dead Zone : DeadZone  LowerValue=-0.005  UpperValue=0.005  SaturateOnIntegerOverflow=on
  Divide : Product  Inputs=*/
  Fb : Product  Inputs=**
  Gain : Gain  Gain=-1/(RBD-VBD)
  Gain1 : Gain  Gain=-1
  Gain3 : Gain  Gain=-1
  Gravity : Gain  Gain=9.81
  Product : Product
  Rate Limiter : RateLimiter  RisingSlewLimit=1/tf  FallingSlewLimit=-1/tl  SampleTimeMode=inherited
  Relational Operator : RelationalOperator  OutDataTypeStr=boolean  RndMeth=Simplest
  Saturation : Saturate  UpperLimit=1  LowerLimit=0
  Saturation Dynamic : simulink/Discontinuities/Saturation Dynamic  OutMin=[]  OutMax=[]  OutDataTypeStr=Inherit: Same as second input  OutDataType=fixdt(1, 16)  OutScaling=2^-10  DoSatur=off
  Strahl formula : Polyval  Coefs=Pres
  Sum1 : Sum  Inputs=|+-
  Switch{,1..4} (5 alike) : Switch  Criteria=u2 ~= 0
  Transfer Fcn : TransferFcn  Numerator=BPnum  Denominator=BPden
  Transport Delay : TransportDelay  DelayTime=l/c  InitialOutput=p0
  efficiency : Product  Inputs=**
  friction coefficient : Constant  Value=fc
  lookup wagon braking efficiency : LookupNDDirect  TableIsInput=on
  lookup wagon mass : LookupNDDirect  TableIsInput=on
  max. braking force before slip : Product  Inputs=**
  "random index, generate once " : commrandsrc3/Random Integer Generator  SetSize=500  SeedSource=Auto  Seed=0  SampleTime=999999  SamplesPerFrame=1  OutputDataType=uint32  SimulateUsing=Interpreted execution
  track gradient : Bias  Bias=9.81*sin(trackgradient)
  v = v0 + a * t : Integrator  InitialConditionSource=external  InitialCondition=v0
  Fres : Outport  VectorParamsAs1DForOutWhenUnconnected=off
  p_BP_out : Outport  Port=2  VectorParamsAs1DForOutWhenUnconnected=off
  ares : Outport  Port=3
  m : Outport  Port=4
  "id " : Outport  Port=5
  wires:
  Strahl formula/1 -> Gravity/1
  Abs/1 -> Strahl formula/1
  Gravity/1 -> Product/2
  Product/1 -> Sum1/2  "Fw"
  v = v0 + a * t/1 -> Abs/1  "v"
  lookup wagon mass/1 -> Gain1/1, Switch3/1, max. braking force before slip/2, Divide/2, Product/1
  Divide/1 -> track gradient/1  "a"
  Gain/1 -> Saturation/1
  Fb/1 -> efficiency/2
  Saturation/1 -> Rate Limiter/1
  Rate Limiter/1 -> Fb/1
  Transfer Fcn/1 -> Dead Zone/1
  Transport Delay/1 -> Transfer Fcn/1
  efficiency/1 -> Sum1/1
  track gradient/1 -> Switch2/1, v = v0 + a * t/1  "ares"
  p/1 -> Gain/1, Transport Delay/1
  friction coefficient/1 -> max. braking force before slip/1
  Sum1/1 -> Saturation Dynamic/2  "Fres"
  Saturation Dynamic/1 -> Switch1/1, Divide/1
  max. braking force before slip/1 -> Saturation Dynamic/1, Gain3/1
  Gain3/1 -> Saturation Dynamic/3
  Data Store Read/1 -> v = v0 + a * t/2
  Dead Zone/1 -> Switch4/1
  Constant/1 -> lookup wagon braking efficiency/3, lookup wagon mass/3
  "random index, generate once "/1 -> Switch/1, lookup wagon mass/1, lookup wagon braking efficiency/1
  Constant1/1 -> lookup wagon mass/2
  Constant2/1 -> lookup wagon braking efficiency/2
  lookup wagon braking efficiency/1 -> efficiency/1
  Gain1/1 -> Fb/2
  Constant3/1 -> Relational Operator/1
  Constant4/1 -> Relational Operator/2
  Relational Operator/1 -> Switch1/2, Switch4/2, Switch2/2, Switch3/2, Switch/2
  Switch/1 -> "id "/1
  Constant5/1 -> Switch4/3, Switch1/3, Switch/3, Switch2/3, Switch3/3
  Switch1/1 -> Fres/1
  Switch2/1 -> ares/1
  Switch3/1 -> m/1
  Switch4/1 -> p_BP_out/1
